simulink model "labview_control_loop_v1"  (R2013a)
settings: Solver=ode45  StartTime=0.0  StopTime=10.0  RelTol=1e-3
libraries: simulink x1
settings Model: Creator=mainster  LastModifiedBy=mainster

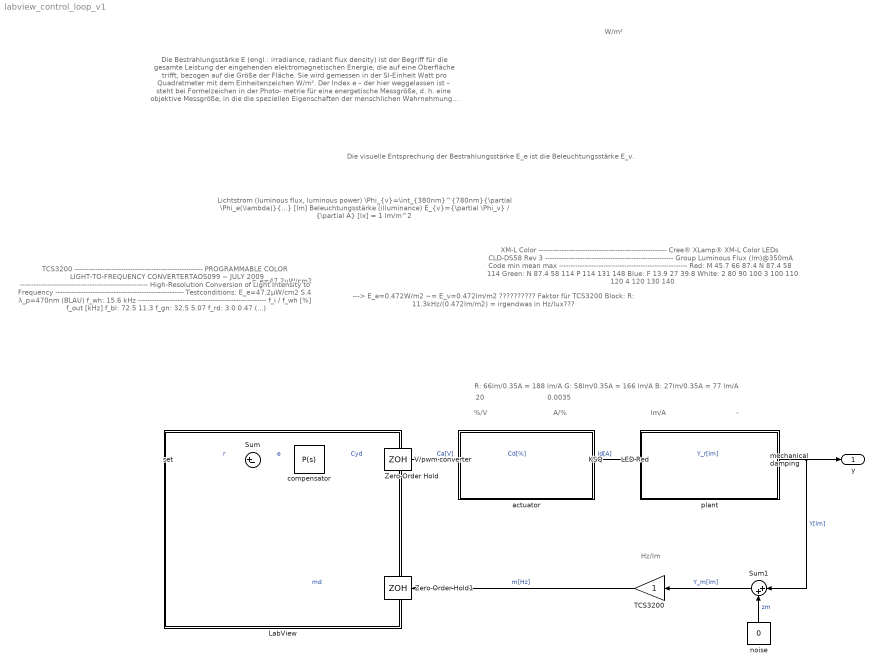
== system labview_control_loop_v1 ==
  note: Die visuelle Entsprechung der Bestrahlungsstärke E_e ist die Beleuchtungsstärke E_v.
  note: W/m²
  note: E_e=47.2µW/cm2
  note: Die Bestrahlungsstärke  E  (engl.: irradiance, radiant flux density) ist der Begriff
      | für die gesamte Leistung der eingehenden elektromagnetischen Energie, die auf
      | eine Oberfläche trifft, bezogen auf die Größe der Fläche. Sie wird gemessen in
      | der SI-Einheit Watt pro Quadratmeter mit dem Einheitenzeichen W/m².
      |
      | Der Index e – der hier weggelassen ist – steht bei Formelzeichen in der Photo-
      | metrie für eine energetische Messgröße, d. h. eine objektive Messgröße, in die
      | die speziellen Eigenschaften der menschlichen Wahrnehmung nicht einfließen.
      | Im Gegensatz dazu steht der Index v für eine visuelle Messgröße, in die die
      | subjektiven Eigenschaften des menschlichen Auges einfließen.
      | Im Bereich der Elektrotechnik wird die Bestrahlungsstärke oft synonym mit
      | der Intensität verwendet, letztere bezieht sich jedoch allgemein auf Wellen.
  note: XM-L Color
      | -------------------------------------------------------
      | Cree® XLamp® XM-L Color LEDs
      | CLD-DS58 Rev 3
      | -------------------------------------------------------
      | Group  	Luminous Flux (lm)@350mA
      | Code	 			min	   mean	max
      | -------------------------------------------------------
      | Red:		M		45.7		66		87.4
      | 			N 		87.4 		58		114
      | Green:	N 		87.4 		58		114
      | 			P 		114 		131	148
      | Blue:		F 		13.9 		27		39.8
      | White:		2 		80 			90 		100
      | 			3 		100 		110	120
      | 			4 		120 		130	140
  note: Lichtstrom
      | (luminous flux,
      | luminous power)		\Phi_{v}=\int_{380nm}^{780nm}{\partial \Phi_e(\lambda)}{...}	[lm]
      | Beleuchtungsstärke
      | (illuminance)				E_{v}={\partial \Phi_v} / {\partial A}	[lx] = 1 lm/m^2
  note: %/V
  note: A/%
  note: lm/A
  note: -
  note: Hz/lm
  note: 20
  note: 0.0035
  note: R:	66lm/0.35A = 188 lm/A
      | G:	58lm/0.35A = 166 lm/A
      | B:	27lm/0.35A = 77 lm/A
  note: TCS3200
      | -------------------------------------------------------
      | PROGRAMMABLE
      | COLOR LIGHT-TO-FREQUENCY
      | CONVERTERTAOS099 − JULY 2009
      | -------------------------------------------------------
      | High-Resolution Conversion of Light
      | Intensity to Frequency
      | -------------------------------------------------------
      | Testconditions:	E_e=47.2µW/cm2
      | S.4					λ_p=470nm (BLAU)
      |
      | f_wh:	  15.6	kHz
      | -------------------------------------------------------
      | 		f_i / f_wh [%]		f_out [kHz]
      | f_bl:		72.5				11.3
      | f_gn:		32.5				5.07
      | f_rd:		  3.0				0.47
      |
      | (...)
  note: ---> E_e=0.472W/m2  ~=  E_v=0.472lm/m2
      | ??????????
      | Faktor für TCS3200 Block:
      |
      | R:	11.3kHz/(0.472lm/m2) = irgendwas in Hz/lux???
  set : Inport
  KSQ : Gain  Gain=0.0035
  LED Red : Gain  Gain=188
  LabView : Subsystem
      mask Display: disp('')
  Sum : Sum  Inputs=|+-
  Sum1 : Sum  Inputs=|++
  TCS3200 : Gain
  V/pwm converter : Gain  Gain=20
  Zero-Order Hold : ZeroOrderHold
  Zero-Order Hold1 : ZeroOrderHold
  actuator : Subsystem
      mask Display: disp('')
  compensator : simulink/Continuous/PID Controller  Controller=P  TimeDomain=Continuous-time  SampleTime=1  IntegratorMethod=Forward Euler  FilterMethod=Forward Euler  Form=Parallel  P=1  I=1  D=0  N=100  InitialConditionSource=internal  InitialConditionForIntegrator=0  InitialConditionForFilter=0  ExternalReset=none  LimitOutput=off  UpperSaturationLimit=inf  LowerSaturationLimit=-inf  LinearizeAsGain=on  AntiWindupMode=none  Kb=1  TrackingMode=off  Kt=1  PParamMin=[]  PParamMax=[]  IParamMin=[]  IParamMax=[]  DParamMin=[]  DParamMax=[]  NParamMin=[]  NParamMax=[]  KbParamMin=[]  KbParamMax=[]  KtParamMin=[]  KtParamMax=[]  POutMin=[]  POutMax=[]  IOutMin=[]  IOutMax=[]  DOutMin=[]  DOutMax=[]  NOutMin=[]  NOutMax=[]  KbOutMin=[]  KbOutMax=[]  KtOutMin=[]  KtOutMax=[]  IntegratorOutMin=[]  IntegratorOutMax=[]  FilterOutMin=[]  FilterOutMax=[]  SumOutMin=[]  SumOutMax=[]  SumI1OutMin=[]  SumI1OutMax=[]  SumI2OutMin=[]  SumI2OutMax=[]  SumI3OutMin=[]  SumI3OutMax=[]  SumDOutMin=[]  SumDOutMax=[]  SaturationOutMin=[]  SaturationOutMax=[]  IntegratorContinuousStateAttributes=''  IntegratorStateMustResolveToSignalObject=off  IntegratorRTWStateStorageClass=Auto  FilterContinuousStateAttributes=''  FilterStateMustResolveToSignalObject=off  FilterRTWStateStorageClass=Auto  mask(PID 1dof){}
      mask Display:
      | % This is a new mask on top of the base mask.
      | % Use "View base mask" link below to see the base mask.
      | fprintf('C(s)\nP/PI')
  mechanical damping : Gain  Gain=0.95
  noise : Constant  Value=0
  plant : Subsystem
      mask Display: disp('')
  y : Outport
  wires:
  Sum/1 -> compensator/1  "e"
  compensator/1 -> Zero-Order Hold/1  "Cyd"
  Zero-Order Hold/1 -> V/pwm converter/1  "Ca[V]"
  V/pwm converter/1 -> KSQ/1  "Cd[%]"
  KSQ/1 -> LED Red/1  "Id[A]"
  mechanical damping/1 -> y/1, Sum1/1  "Y[lm]"
  noise/1 -> Sum1/2  "zm"
  Sum1/1 -> TCS3200/1  "Y_m[lm]"
  LED Red/1 -> mechanical damping/1  "Y_r[lm]"
  TCS3200/1 -> Zero-Order Hold1/1  "m[Hz]"
  set/1 -> Sum/1  "r"
  Zero-Order Hold1/1 -> Sum/2  "md"

== system labview_control_loop_v1/LabView ==

== system labview_control_loop_v1/actuator ==

== system labview_control_loop_v1/plant ==
